simulink model "OSQP"  (R2025a)
settings: Solver=ode8  StartTime=0.0  StopTime=10  FixedStep=100e-7  RelTol=1e-3
settings Model: Creator=JR  LastModifiedBy=JR

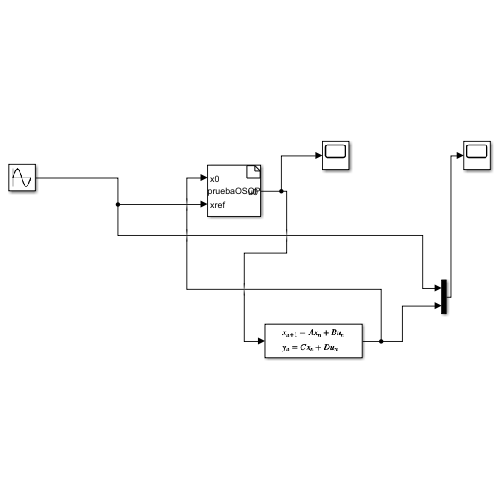
[thumbnail: Simulink's stored preview of the top-level diagram]
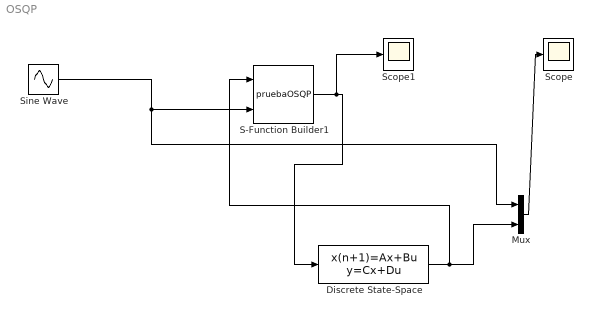
== system OSQP ==
  Discrete State-Space : DiscreteStateSpace  D=0  InitialCondition=2  SampleTime=100e-6
  Mux : Mux  Inputs=2
  S-Function Builder1 : S-Function  FunctionName=pruebaOSQP  SFunctionModules=pruebaOSQP_wrapper.c cpg_workspace cpg_solve workspace emosqp algebra_libs auxil csc_math csc_utils error kkt matrix osqp_api qdldl qdldl_interface scaling util vector  SFunctionDeploymentMode=off  EnableBusSupport=off  mask(S-Function Builder){}
      mask help: Simulink:masks:SFunctionBuilder_MD
      mask init:
      | val = [[.9  0.75 0.75 1 1 .9 .9 1]',[1 1 0.75 0.75 .9 .9 1 .9]'];try , sys = get_param(gcb,'SfunBuilderFcnName');if isempty(sys), sys = get_param(gcb,'FunctionName'); end,catch, sys = get_param(gcb,'FunctionName'); end
      settings: CopyFcn=set_param(gcbh,'LinkStatus','none')  OpenFcn=sfunctionwizard(gcbh)
      mask Display:
      | plot(val(:,1),val(:,2))
      | disp(sys)
      | port_label('input',1,sprintf('%s', 'x0'),'interpreter','tex')
      | port_label('input',2,sprintf('%s', 'xref'),'interpreter','tex')
      | port_label('output',1,sprintf('%s', 'u0'),'interpreter','tex')
  Scope : Scope
      settings: ActiveDisplayYMinimum=-2.4999999999992371  ActiveDisplayYMaximum=2.4999999999999152
  Scope1 : Scope
      settings: ActiveDisplayYMinimum=-0.0022855553558398523  ActiveDisplayYMaximum=0.0010700176669411964
  Sine Wave : Sin  Amplitude=2  Frequency=10  SampleTime=0
  wires:
  Mux/1 -> Scope/1
  S-Function Builder1/1 -> Scope1/1, Discrete State-Space/1
  Discrete State-Space/1 -> S-Function Builder1/1, Mux/2
  Sine Wave/1 -> S-Function Builder1/2, Mux/1
